simulink model "DC_motor_EX1"  (R2022a)
settings: Solver=VariableStepAuto  StartTime=0.0  StopTime=0.2  RelTol=1e-3
values from neighbouring files (symbols this model uses):
  Ad = dis_sys.A    [DC_motor.m]
  B_noise1 = [Bd Bw]    [DC_motor.m]
  Cd = dis_sys.C    [DC_motor.m]
  D_noise1 = [Dd Dd Dd]    [DC_motor.m]
  Ts = 1e-3    (= 0.001)    [DC_motor.m]
  W = [1 ... (first row only)    [DC_motor.m]
  x0 = [I0 n0]'    [DC_motor.m]
undefined symbols (not defined in the file or in its folder): Kdlqr
settings Model: Creator=Shahin  LastModifiedBy=jj
settings SolverCC: AlgebraicLoopSolver=TrustRegion
settings DataIOCC: ReturnWorkspaceOutputs=off
settings DebuggingCC: UnconnectedInputMsg=warning  UnconnectedOutputMsg=warning  UnconnectedLineMsg=warning  SFMachineParentedDataDiag=warning  ArithmeticOperatorsInVariantConditions=warning
settings SFSimCC: CustomCodeUndefinedFunction=UseInterfaceOnly

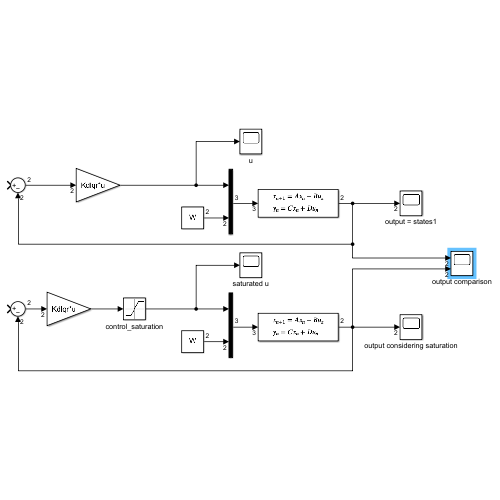
[thumbnail: Simulink's stored preview of the top-level diagram]
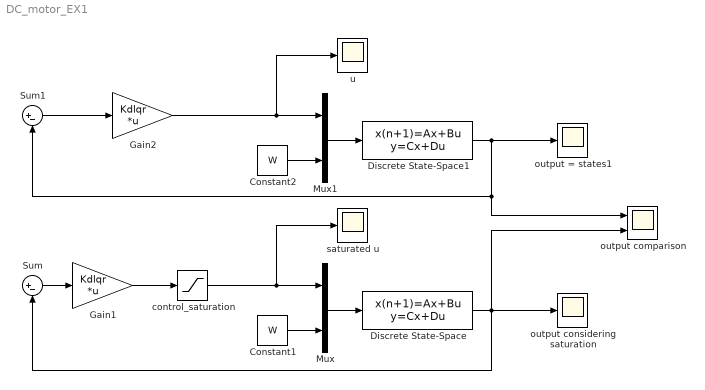
== system DC_motor_EX1 ==
  Constant1 : Constant  Value=W  SampleTime=Ts
  Constant2 : Constant  Value=W  SampleTime=Ts
  Discrete State-Space : DiscreteStateSpace  A=Ad  B=B_noise1  C=Cd  D=D_noise1  InitialCondition=x0  SampleTime=Ts
  Discrete State-Space1 : DiscreteStateSpace  A=Ad  B=B_noise1  C=Cd  D=D_noise1  InitialCondition=x0  SampleTime=Ts
  Gain1 : Gain  Gain=Kdlqr  Multiplication=Matrix(K*u)
  Gain2 : Gain  Gain=Kdlqr  Multiplication=Matrix(K*u)
  Mux : Mux  Inputs=2
  Mux1 : Mux  Inputs=2
  Sum : Sum  Inputs=|+-
  Sum1 : Sum  Inputs=|+-
  control_saturation : Saturate  UpperLimit=12  LowerLimit=0
  output = states1 : Scope
  output comparison : Scope  NumInputPorts=2
  output considering saturation : Scope
  saturated u : Scope
  u : Scope
  wires:
  Mux/1 -> Discrete State-Space/1
  Gain1/1 -> control_saturation/1
  Sum/1 -> Gain1/1
  Discrete State-Space/1 -> output comparison/2, Sum/2, output considering saturation/1
  control_saturation/1 -> saturated u/1, Mux/1
  Constant1/1 -> Mux/2
  Sum1/1 -> Gain2/1
  Mux1/1 -> Discrete State-Space1/1
  Constant2/1 -> Mux1/2
  Gain2/1 -> u/1, Mux1/1
  Discrete State-Space1/1 -> output comparison/1, Sum1/2, output = states1/1
